simulink model "fft_biplex_test3"  (Simulink 7.6)
settings: Solver=ode45  StartTime=0.0  StopTime=5000  RelTol=1e-3
libraries: xbsIndex_r4 x1382, casper_library x82, monroe_library x27, xps_library x17, dspsigops x16, simulink x1
(part 3 of 13)

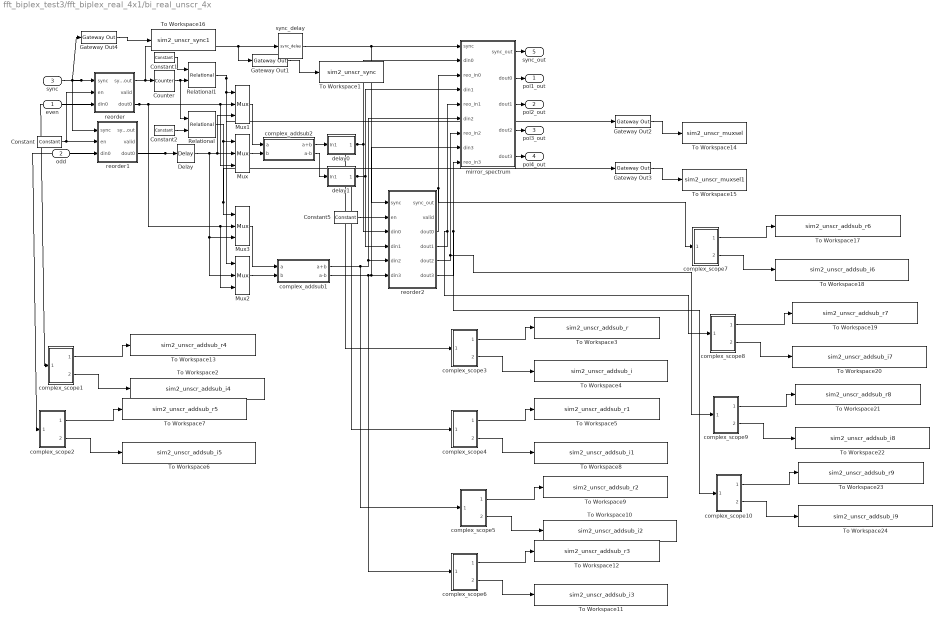
== system fft_biplex_test3/fft_biplex_real_4x1/bi_real_unscr_4x ==
  even : Inport
  odd : Inport  Port=2
  sync : Inport  Port=3
  Constant : xbsIndex_r4/Constant  arith_type=Boolean  const=1  n_bits=1  bin_pt=0  explicit_period=on  period=1  equ=P=C  opselect=C  inp2=PCIN>>17  opr=+  inp1=P  carry=CIN  dbl_ovrd=off  block_type=constant
      settings: block_version=9.1.01
  Constant1 : xbsIndex_r4/Constant  arith_type=Unsigned  const=2^(FFTSize-1)-1  n_bits=FFTSize  bin_pt=0  explicit_period=on  period=1  equ=P=C  opselect=C  inp2=PCIN>>17  opr=+  inp1=P  carry=CIN  dbl_ovrd=off  block_type=constant
      settings: block_version=9.1.01
  Constant2 : xbsIndex_r4/Constant  arith_type=Unsigned  const=2^FFTSize -1  n_bits=FFTSize  bin_pt=0  explicit_period=on  period=1  equ=P=C  opselect=C  inp2=PCIN>>17  opr=+  inp1=P  carry=CIN  dbl_ovrd=off  block_type=constant
      settings: block_version=9.1.01
  Constant5 : xbsIndex_r4/Constant  arith_type=Boolean  const=1  n_bits=1  bin_pt=0  explicit_period=on  period=1  equ=P=C  opselect=C  inp2=PCIN>>17  opr=+  inp1=P  carry=CIN  dbl_ovrd=off  block_type=constant
      settings: block_version=9.1.01
  Counter : xbsIndex_r4/Counter  cnt_type=Free Running  cnt_to=Inf  operation=Up  start_count=0  cnt_by_val=1  arith_type=Unsigned  n_bits=FFTSize  bin_pt=0  load_pin=off  rst=on  en=off  explicit_period=off  period=1  dbl_ovrd=off  use_behavioral_HDL=off  implementation=Fabric  use_rpm=on  block_type=counter
      settings: xl_area=[0, 0, 0, 0, 0, 0, 0]  block_version=9.1.01
  Delay : xbsIndex_r4/Delay  en=off  latency=1  dbl_ovrd=off  reg_retiming=off  block_type=delay
      settings: xl_area=[0, 0, 0, 0, 0, 0, 0]  block_version=9.1.01
  Gateway Out{1..4} (4 alike) : xbsIndex_r4/Gateway Out  hdl_port=on  timing_constraint=None  locs_specified=off  LOCs={}  block_type=gatewayout
      settings: infoedit="Gateway out block.  Converts Xilinx fixed point inputs into ouputs of type Simulink integer, double, or fixed point.<br><br>Hardware notes:  In hardware these blocks become top level output ports or are discarded, depending on how they are configured."  block_version=11.4
  Mux{,1..3} (4 alike) : xbsIndex_r4/Mux  inputs=2  en=off  latency=1  precision=Full  arith_type="Signed  (2's comp)"  n_bits=8  bin_pt=2  quantization=Truncate  overflow=Wrap  dbl_ovrd=off  block_type=mux
      settings: xl_area=[0, 0, 0, 0, 0, 0, 0]  block_version=9.1.01
  Relational : xbsIndex_r4/Relational  mode=a=b  en=off  latency=1  dbl_ovrd=off  block_type=relational
      settings: xl_area=[0, 0, 0, 0, 0, 0, 0]  block_version=9.1.01
  Relational1 : xbsIndex_r4/Relational  mode=a=b  en=off  latency=1  dbl_ovrd=off  block_type=relational
      settings: xl_area=[0, 0, 0, 0, 0, 0, 0]  block_version=9.1.01
  To Workspace1 : ToWorkspace  VariableName=sim2_unscr_sync  SampleTime=-1  SaveFormat=Structure
  To Workspace10 : ToWorkspace  VariableName=sim2_unscr_addsub_i2  SampleTime=-1  SaveFormat=Structure
  To Workspace11 : ToWorkspace  VariableName=sim2_unscr_addsub_i3  SampleTime=-1  SaveFormat=Structure
  To Workspace12 : ToWorkspace  VariableName=sim2_unscr_addsub_r3  SampleTime=-1  SaveFormat=Structure
  To Workspace13 : ToWorkspace  VariableName=sim2_unscr_addsub_r4  SampleTime=-1  SaveFormat=Structure
  To Workspace14 : ToWorkspace  VariableName=sim2_unscr_muxsel  SampleTime=-1  SaveFormat=Structure
  To Workspace15 : ToWorkspace  VariableName=sim2_unscr_muxsel1  SampleTime=-1  SaveFormat=Structure
  To Workspace16 : ToWorkspace  VariableName=sim2_unscr_sync1  SampleTime=-1  SaveFormat=Structure
  To Workspace17 : ToWorkspace  VariableName=sim2_unscr_addsub_r6  SampleTime=-1  SaveFormat=Structure
  To Workspace18 : ToWorkspace  VariableName=sim2_unscr_addsub_i6  SampleTime=-1  SaveFormat=Structure
  To Workspace19 : ToWorkspace  VariableName=sim2_unscr_addsub_r7  SampleTime=-1  SaveFormat=Structure
  To Workspace2 : ToWorkspace  VariableName=sim2_unscr_addsub_i4  SampleTime=-1  SaveFormat=Structure
  To Workspace20 : ToWorkspace  VariableName=sim2_unscr_addsub_i7  SampleTime=-1  SaveFormat=Structure
  To Workspace21 : ToWorkspace  VariableName=sim2_unscr_addsub_r8  SampleTime=-1  SaveFormat=Structure
  To Workspace22 : ToWorkspace  VariableName=sim2_unscr_addsub_i8  SampleTime=-1  SaveFormat=Structure
  To Workspace23 : ToWorkspace  VariableName=sim2_unscr_addsub_r9  SampleTime=-1  SaveFormat=Structure
  To Workspace24 : ToWorkspace  VariableName=sim2_unscr_addsub_i9  SampleTime=-1  SaveFormat=Structure
  To Workspace3 : ToWorkspace  VariableName=sim2_unscr_addsub_r  SampleTime=-1  SaveFormat=Structure
  To Workspace4 : ToWorkspace  VariableName=sim2_unscr_addsub_i  SampleTime=-1  SaveFormat=Structure
  To Workspace5 : ToWorkspace  VariableName=sim2_unscr_addsub_r1  SampleTime=-1  SaveFormat=Structure
  To Workspace6 : ToWorkspace  VariableName=sim2_unscr_addsub_i5  SampleTime=-1  SaveFormat=Structure
  To Workspace7 : ToWorkspace  VariableName=sim2_unscr_addsub_r5  SampleTime=-1  SaveFormat=Structure
  To Workspace8 : ToWorkspace  VariableName=sim2_unscr_addsub_i1  SampleTime=-1  SaveFormat=Structure
  To Workspace9 : ToWorkspace  VariableName=sim2_unscr_addsub_r2  SampleTime=-1  SaveFormat=Structure
  complex_addsub1 : Subsystem  mask(complex_addsub){BitWidth=input_bit_width, add_latency=add_latency}
      mask prompts: BitWidth "Bit Wdith"; add_latency "Add Latency"
      mask help:
      | Adds and subtracts the complex inputs.
      | If a = w + ix, b = y + iz then
      | a+b = (w+y)/2 + i(x-z)/2 and
      | a-b = (x+z)/2 + i(y-w)/2
  complex_addsub2 : Subsystem  mask(complex_addsub){BitWidth=input_bit_width, add_latency=add_latency}
      mask prompts: BitWidth "Bit Wdith"; add_latency "Add Latency"
      mask help:
      | Adds and subtracts the complex inputs.
      | If a = w + ix, b = y + iz then
      | a+b = (w+y)/2 + i(x-z)/2 and
      | a-b = (x+z)/2 + i(y-w)/2
  complex_scope1 : Subsystem
  complex_scope10 : Subsystem
  complex_scope2 : Subsystem
  complex_scope3 : Subsystem
  complex_scope4 : Subsystem
  complex_scope5 : Subsystem
  complex_scope6 : Subsystem
  complex_scope7 : Subsystem
  complex_scope8 : Subsystem
  complex_scope9 : Subsystem
  delay0 : Subsystem  AncestorBlock=casper_library/Delays/delay_bram  mask(delay_bram){DelayLen=2^(FFTSize-1), bram_latency=bram_latency, use_dsp48=off}
      mask prompts: DelayLen "Delay By:"; bram_latency "BRAM Latency"; use_dsp48 "Use DSP48"
      mask help: A delay block that uses BRAM for its storage.
      mask init:
      | if (DelayLen <= bram_latency)
      | 	error('delay value must be greater than BRAM Latency');
      | end
      | BitWidth = max(ceil(log2(DelayLen)), 2);
      | if strcmp(use_dsp48,'on'),
      |     set_param([gcb,'/Counter'], 'use_behavioral_HDL', 'off', ...
      |         'use_rpm', 'on', 'implementation', 'DSP48');
      | else, %default counter settings
      |         set_param([gcb,'/Counter'], 'use_behavioral_HDL', 'off', ...
      |         'use_rpm', 'off', 'implementation', 'Fabric');
      | end
      mask Help: eval('xlWeb(''http://casper.berkeley.edu/wiki/Delay_bram'')')
  delay1 : Subsystem  AncestorBlock=casper_library/Delays/delay_bram  mask(delay_bram){DelayLen=2^(FFTSize-1), bram_latency=bram_latency, use_dsp48=off}
      mask prompts: DelayLen "Delay By:"; bram_latency "BRAM Latency"; use_dsp48 "Use DSP48"
      mask help: A delay block that uses BRAM for its storage.
      mask init: same as fft_biplex_test3/fft_biplex_real_4x1/bi_real_unscr_4x/delay0
      mask Help: eval('xlWeb(''http://casper.berkeley.edu/wiki/Delay_bram'')')
  mirror_spectrum : Subsystem
  reorder : Subsystem  AncestorBlock=casper_library/Reorder/reorder  mask(reorder){map=getfield( getfield( get_param( gcb,'UserData' ), 'parameters'),'map'), n_inputs=1, bram_latency=3, map_latency=0, double_buffer=0}
      mask prompts: map "Output Order:"; n_inputs "Number of inputs"; bram_latency "BRAM Latency"; map_latency "Map Latency"; double_buffer "Double Buffer"
      mask init:
      | reorder_init(gcb, ...
      |     'map', map, ...
      |     'n_inputs', n_inputs, ...
      |     'bram_latency', bram_latency, ...
      |     'map_latency', map_latency, ...
      |     'double_buffer', double_buffer);
      settings: AttributesFormatString=order=2
  reorder1 : Subsystem  AncestorBlock=casper_library/Reorder/reorder  mask(reorder){map=getfield( getfield( get_param( gcb,'UserData' ), 'parameters'),'map'), n_inputs=1, bram_latency=3, map_latency=0, double_buffer=0}
      mask prompts: map "Output Order:"; n_inputs "Number of inputs"; bram_latency "BRAM Latency"; map_latency "Map Latency"; double_buffer "Double Buffer"
      mask init:
      | reorder_init(gcb, ...
      |     'map', map, ...
      |     'n_inputs', n_inputs, ...
      |     'bram_latency', bram_latency, ...
      |     'map_latency', map_latency, ...
      |     'double_buffer', double_buffer);
      settings: AttributesFormatString=order=2
  reorder2 : Subsystem  AncestorBlock=casper_library/Reorder/reorder  mask(reorder){map=getfield( getfield( get_param( gcb,'UserData' ), 'parameters'),'map'), n_inputs=4, bram_latency=3, map_latency=0, double_buffer=0}
      mask prompts: map "Output Order:"; n_inputs "Number of inputs"; bram_latency "BRAM Latency"; map_latency "Map Latency"; double_buffer "Double Buffer"
      mask init:
      | reorder_init(gcb, ...
      |     'map', map, ...
      |     'n_inputs', n_inputs, ...
      |     'bram_latency', bram_latency, ...
      |     'map_latency', map_latency, ...
      |     'double_buffer', double_buffer);
      settings: AttributesFormatString=order=2
  sync_delay : casper_library/Delays/sync_delay  SystemSampleTime=-1  DelayLen=2^(FFTSize-1) + 2*add_latency+1
  pol1_out : Outport
  pol2_out : Outport  Port=2
  pol3_out : Outport  Port=3
  pol4_out : Outport  Port=4
  sync_out : Outport  Port=5
  wires:
  reorder2/6(dout3) -> mirror_spectrum/9(reo_in3), complex_scope10/1(In1)
  reorder2/5(dout2) -> mirror_spectrum/7(reo_in2), complex_scope9/1(In1)
  reorder2/3(dout0) -> mirror_spectrum/3(reo_in0), complex_scope7/1(In1)
  reorder2/4(dout1) -> mirror_spectrum/5(reo_in1), complex_scope8/1(In1)
  mirror_spectrum/2(dout0) -> pol1_out/1
  mirror_spectrum/1(sync_out) -> sync_out/1
  sync_delay/1 -> mirror_spectrum/1(sync), reorder2/1(sync)
  Constant5/1 -> reorder2/2(en)
  delay0/1(Out1) -> mirror_spectrum/2(din0), reorder2/3(din0), complex_scope3/1(In1)
  delay1/1(Out1) -> mirror_spectrum/4(din1), reorder2/4(din1), complex_scope4/1(In1)
  complex_addsub1/1(a+b) -> mirror_spectrum/6(din2), reorder2/5(din2), complex_scope5/1(In1)
  complex_addsub1/2(a-b) -> mirror_spectrum/8(din3), reorder2/6(din3), complex_scope6/1(In1)
  complex_addsub2/2(a-b) -> delay1/1(In1)
  complex_addsub2/1(a+b) -> delay0/1(In1)
  Mux3/1 -> complex_addsub1/1(a)
  Mux2/1 -> complex_addsub1/2(b)
  Relational1/1 -> Mux1/1, Mux2/1, Gateway Out2/1
  Constant1/1 -> Relational1/1
  Counter/1 -> Relational1/2, Relational/1
  Constant2/1 -> Relational/2
  Mux1/1 -> complex_addsub2/1(a)
  sync/1 -> reorder1/1(sync), reorder/1(sync), Gateway Out4/1
  Constant/1 -> reorder1/2(en), reorder/2(en)
  reorder1/3(dout0) -> Delay/1, complex_scope2/1(In1)
  reorder/3(dout0) -> Mux3/2, Mux2/3, Mux1/2, Mux/3, complex_scope1/1(In1)
  reorder/1(sync_out) -> Counter/1, sync_delay/1, Gateway Out1/1
  Delay/1 -> Mux1/3, Mux/2, Mux3/3, Mux2/2
  Mux/1 -> complex_addsub2/2(b)
  Relational/1 -> Mux/1, Mux3/1, Gateway Out3/1
  even/1 -> reorder/3(din0)
  odd/1 -> reorder1/3(din0)
  mirror_spectrum/3(dout1) -> pol2_out/1
  mirror_spectrum/4(dout2) -> pol3_out/1
  mirror_spectrum/5(dout3) -> pol4_out/1
  complex_scope3/1(Real) -> To Workspace3/1
  complex_scope3/2(Imag) -> To Workspace4/1
  complex_scope4/1(Real) -> To Workspace5/1
  complex_scope4/2(Imag) -> To Workspace8/1
  complex_scope5/1(Real) -> To Workspace9/1
  complex_scope5/2(Imag) -> To Workspace10/1
  complex_scope6/1(Real) -> To Workspace12/1
  complex_scope6/2(Imag) -> To Workspace11/1
  Gateway Out1/1 -> To Workspace1/1
  Gateway Out2/1 -> To Workspace14/1
  Gateway Out3/1 -> To Workspace15/1
  Gateway Out4/1 -> To Workspace16/1
  complex_scope1/1(Real) -> To Workspace13/1
  complex_scope1/2(Imag) -> To Workspace2/1
  complex_scope2/1(Real) -> To Workspace7/1
  complex_scope2/2(Imag) -> To Workspace6/1
  complex_scope7/1(Real) -> To Workspace17/1
  complex_scope7/2(Imag) -> To Workspace18/1
  complex_scope8/1(Real) -> To Workspace19/1
  complex_scope8/2(Imag) -> To Workspace20/1
  complex_scope9/1(Real) -> To Workspace21/1
  complex_scope9/2(Imag) -> To Workspace22/1
  complex_scope10/1(Real) -> To Workspace23/1
  complex_scope10/2(Imag) -> To Workspace24/1

== system fft_biplex_test3/fft_biplex_real_4x1/biplex_core ==
  pol1 : Inport
  pol2 : Inport  Port=2
  sync : Inport  Port=3
  shift : Inport  Port=4
  Constant : xbsIndex_r4/Constant  arith_type=Boolean  const=0  n_bits=1  bin_pt=1  explicit_period=off  period=1  equ=P=C  opselect=C  inp2=PCIN>>17  opr=+  inp1=P  carry=CIN  dbl_ovrd=off  block_type=constant
  To Workspace1 : ToWorkspace  VariableName=sim2_stg4_r  SampleTime=-1  SaveFormat=Structure
  To Workspace10 : ToWorkspace  VariableName=sim2_stg3_r  SampleTime=-1  SaveFormat=Structure
  To Workspace11 : ToWorkspace  VariableName=sim2_stg3_i  SampleTime=-1  SaveFormat=Structure
  To Workspace12 : ToWorkspace  VariableName=sim2_stg2_i1  SampleTime=-1  SaveFormat=Structure
  To Workspace2 : ToWorkspace  VariableName=sim2_stg4_i  SampleTime=-1  SaveFormat=Structure
  To Workspace3 : ToWorkspace  VariableName=sim2_stg4_r1  SampleTime=-1  SaveFormat=Structure
  To Workspace4 : ToWorkspace  VariableName=sim2_stg3_r1  SampleTime=-1  SaveFormat=Structure
  To Workspace5 : ToWorkspace  VariableName=sim2_stg3_i1  SampleTime=-1  SaveFormat=Structure
  To Workspace6 : ToWorkspace  VariableName=sim2_stg4_i1  SampleTime=-1  SaveFormat=Structure
  To Workspace7 : ToWorkspace  VariableName=sim2_stg2_r  SampleTime=-1  SaveFormat=Structure
  To Workspace8 : ToWorkspace  VariableName=sim2_stg2_i  SampleTime=-1  SaveFormat=Structure
  To Workspace9 : ToWorkspace  VariableName=sim2_stg2_r1  SampleTime=-1  SaveFormat=Structure
  complex_scope1 : Subsystem
  complex_scope2 : Subsystem
  complex_scope3 : Subsystem
  complex_scope4 : Subsystem
  complex_scope5 : Subsystem
  complex_scope6 : Subsystem
  fft_stage_1 : Subsystem  AncestorBlock=casper_library/FFTs/fft_stage_n  mask(fft_stage_n){FFTSize=5, FFTStage=1, input_bit_width=8, coeff_bit_width=18, delays_bram=on, coeffs_bram=off, MaxCoeffNum=20, quantization=Truncate, overflow=Wrap, add_latency=2, mult_latency=3, bram_latency=3, arch=Virtex5, opt_target=Logic, use_hdl=on, use_embedded=off, dsp48_adders=on, shift=1, output_bit_width=18}
      mask prompts: FFTSize "Size of FFT: (2^? pnts)"; FFTStage "Stage of FFT:"; input_bit_width "Input Bit Width:"; coeff_bit_width "Coefficient Bit Width"; delays_bram "Implement Delays in BRAM:"; coeffs_bram "Store Coefficients in BRAM:"; MaxCoeffNum "Maximum Coefficient Depth: (2^?)"; quantization "Quantization Behavior"; overflow "Overflow Behavior"; add_latency "Add Latency"; mult_latency "Mult Latency"; bram_latency "BRAM Latency"; arch "Architecture"; opt_target "Optimisation target"; use_hdl "Use behavioural HDL for mutlipliers"; use_embedded "Use embedded multipliers"; dsp48_adders "Use DSP48s for adders"; shift "Downshift binary point?"; output_bit_width "Output Bit Width"
      mask init:
      | fft_stage_n_init(gcb,...
      |     'FFTSize', FFTSize,...
      |     'FFTStage', FFTStage,...
      |     'input_bit_width', input_bit_width,...
      |     'output_bit_width', output_bit_width,...
      |     'coeff_bit_width', coeff_bit_width,...
      |     'delays_bram', delays_bram,...
      |     'coeffs_bram', coeffs_bram,...
      |     'MaxCoeffNum', MaxCoeffNum,...
      |     'quantization', quantization,...
      |     'overflow', overflow,...
      |     'add_latency', add_latency,...
      |     'mult_latency', mult_latency,...
      |     'bram_latency', bram_latency,...
      |     'arch', arch, ...
      |     'opt_target', opt_target, ...
      |     'use_hdl', use_hdl,...
      |     'use_embedded', use_embedded, ...
      |     'dsp48_adders', dsp48_adders, ...
      |     'output_bit_width', output_bit_width, ...
      |     'shift', shift );
      settings: AttributesFormatString=|
      | FFTSize=5, FFTStage=1,
      |  coeffs_bram=off,
      |  delays_bram=on
      mask StyleString: edit,edit,edit,edit,checkbox,checkbox,edit,popup(Truncate|Round  (unbiased: +/- Inf)|Round  (unbiased: Even Values)),popup(Wrap|Saturate|Error),edit,edit,edit,popup(Virtex2Pro|Virtex5),popup(Logic|Multipliers),checkbox,checkbox,checkbox,edit,edit
      mask CallbackString:
      | ||||||||||||||use_hdl = get_param(gcb,'use_hdl');
      | visibs = get_param(gcb, 'MaskVisibilities');
      | if( strcmp(use_hdl,'on')),
      |     visibs{16} = 'off';
      | else,
      |     visibs{16} = 'on';
      | end
      |     set_param(gcb, 'MaskVisibilities',visibs);||||
  fft_stage_2 : Subsystem  AncestorBlock=casper_library/FFTs/fft_stage_n  mask(fft_stage_n){FFTSize=5, FFTStage=2, input_bit_width=18, coeff_bit_width=18, delays_bram=on, coeffs_bram=off, MaxCoeffNum=20, quantization=Truncate, overflow=Wrap, add_latency=2, mult_latency=3, bram_latency=3, arch=Virtex5, opt_target=Logic, use_hdl=on, use_embedded=off, dsp48_adders=on, shift=1, output_bit_width=18}
      mask prompts: FFTSize "Size of FFT: (2^? pnts)"; FFTStage "Stage of FFT:"; input_bit_width "Input Bit Width:"; coeff_bit_width "Coefficient Bit Width"; delays_bram "Implement Delays in BRAM:"; coeffs_bram "Store Coefficients in BRAM:"; MaxCoeffNum "Maximum Coefficient Depth: (2^?)"; quantization "Quantization Behavior"; overflow "Overflow Behavior"; add_latency "Add Latency"; mult_latency "Mult Latency"; bram_latency "BRAM Latency"; arch "Architecture"; opt_target "Optimisation target"; use_hdl "Use behavioural HDL for mutlipliers"; use_embedded "Use embedded multipliers"; dsp48_adders "Use DSP48s for adders"; shift "Downshift binary point?"; output_bit_width "Output Bit Width"
      mask init: same as fft_biplex_test3/fft_biplex_real_4x1/biplex_core/fft_stage_1
      settings: AttributesFormatString=|
      | FFTSize=5, FFTStage=2,
      |  coeffs_bram=off,
      |  delays_bram=on
      mask StyleString: edit,edit,edit,edit,checkbox,checkbox,edit,popup(Truncate|Round  (unbiased: +/- Inf)|Round  (unbiased: Even Values)),popup(Wrap|Saturate|Error),edit,edit,edit,popup(Virtex2Pro|Virtex5),popup(Logic|Multipliers),checkbox,checkbox,checkbox,edit,edit
      mask CallbackString:
      | ||||||||||||||use_hdl = get_param(gcb,'use_hdl');
      | visibs = get_param(gcb, 'MaskVisibilities');
      | if( strcmp(use_hdl,'on')),
      |     visibs{16} = 'off';
      | else,
      |     visibs{16} = 'on';
      | end
      |     set_param(gcb, 'MaskVisibilities',visibs);||||
  fft_stage_3 : Subsystem  AncestorBlock=casper_library/FFTs/fft_stage_n  mask(fft_stage_n){FFTSize=5, FFTStage=3, input_bit_width=18, coeff_bit_width=18, delays_bram=off, coeffs_bram=off, MaxCoeffNum=20, quantization=Truncate, overflow=Wrap, add_latency=2, mult_latency=3, bram_latency=3, arch=Virtex5, opt_target=Logic, use_hdl=on, use_embedded=off, dsp48_adders=on, shift=1, output_bit_width=18}
      mask prompts: FFTSize "Size of FFT: (2^? pnts)"; FFTStage "Stage of FFT:"; input_bit_width "Input Bit Width:"; coeff_bit_width "Coefficient Bit Width"; delays_bram "Implement Delays in BRAM:"; coeffs_bram "Store Coefficients in BRAM:"; MaxCoeffNum "Maximum Coefficient Depth: (2^?)"; quantization "Quantization Behavior"; overflow "Overflow Behavior"; add_latency "Add Latency"; mult_latency "Mult Latency"; bram_latency "BRAM Latency"; arch "Architecture"; opt_target "Optimisation target"; use_hdl "Use behavioural HDL for mutlipliers"; use_embedded "Use embedded multipliers"; dsp48_adders "Use DSP48s for adders"; shift "Downshift binary point?"; output_bit_width "Output Bit Width"
      mask init: same as fft_biplex_test3/fft_biplex_real_4x1/biplex_core/fft_stage_1
      settings: AttributesFormatString=|
      | FFTSize=5, FFTStage=3,
      |  coeffs_bram=off,
      |  delays_bram=off
      mask StyleString: edit,edit,edit,edit,checkbox,checkbox,edit,popup(Truncate|Round  (unbiased: +/- Inf)|Round  (unbiased: Even Values)),popup(Wrap|Saturate|Error),edit,edit,edit,popup(Virtex2Pro|Virtex5),popup(Logic|Multipliers),checkbox,checkbox,checkbox,edit,edit
      mask CallbackString:
      | ||||||||||||||use_hdl = get_param(gcb,'use_hdl');
      | visibs = get_param(gcb, 'MaskVisibilities');
      | if( strcmp(use_hdl,'on')),
      |     visibs{16} = 'off';
      | else,
      |     visibs{16} = 'on';
      | end
      |     set_param(gcb, 'MaskVisibilities',visibs);||||
  fft_stage_4 : Subsystem  AncestorBlock=casper_library/FFTs/fft_stage_n  mask(fft_stage_n){FFTSize=5, FFTStage=4, input_bit_width=18, coeff_bit_width=18, delays_bram=off, coeffs_bram=off, MaxCoeffNum=20, quantization=Truncate, overflow=Wrap, add_latency=2, mult_latency=3, bram_latency=3, arch=Virtex5, opt_target=Logic, use_hdl=on, use_embedded=off, dsp48_adders=on, shift=1, output_bit_width=18}
      mask prompts: FFTSize "Size of FFT: (2^? pnts)"; FFTStage "Stage of FFT:"; input_bit_width "Input Bit Width:"; coeff_bit_width "Coefficient Bit Width"; delays_bram "Implement Delays in BRAM:"; coeffs_bram "Store Coefficients in BRAM:"; MaxCoeffNum "Maximum Coefficient Depth: (2^?)"; quantization "Quantization Behavior"; overflow "Overflow Behavior"; add_latency "Add Latency"; mult_latency "Mult Latency"; bram_latency "BRAM Latency"; arch "Architecture"; opt_target "Optimisation target"; use_hdl "Use behavioural HDL for mutlipliers"; use_embedded "Use embedded multipliers"; dsp48_adders "Use DSP48s for adders"; shift "Downshift binary point?"; output_bit_width "Output Bit Width"
      mask init: same as fft_biplex_test3/fft_biplex_real_4x1/biplex_core/fft_stage_1
      settings: AttributesFormatString=|
      | FFTSize=5, FFTStage=4,
      |  coeffs_bram=off,
      |  delays_bram=off
      mask StyleString: edit,edit,edit,edit,checkbox,checkbox,edit,popup(Truncate|Round  (unbiased: +/- Inf)|Round  (unbiased: Even Values)),popup(Wrap|Saturate|Error),edit,edit,edit,popup(Virtex2Pro|Virtex5),popup(Logic|Multipliers),checkbox,checkbox,checkbox,edit,edit
      mask CallbackString:
      | ||||||||||||||use_hdl = get_param(gcb,'use_hdl');
      | visibs = get_param(gcb, 'MaskVisibilities');
      | if( strcmp(use_hdl,'on')),
      |     visibs{16} = 'off';
      | else,
      |     visibs{16} = 'on';
      | end
      |     set_param(gcb, 'MaskVisibilities',visibs);||||
  fft_stage_5 : Subsystem  AncestorBlock=casper_library/FFTs/fft_stage_n  mask(fft_stage_n){FFTSize=5, FFTStage=5, input_bit_width=18, coeff_bit_width=18, delays_bram=off, coeffs_bram=off, MaxCoeffNum=20, quantization=Truncate, overflow=Wrap, add_latency=2, mult_latency=3, bram_latency=3, arch=Virtex5, opt_target=Logic, use_hdl=on, use_embedded=off, dsp48_adders=on, shift=1, output_bit_width=18}
      mask prompts: FFTSize "Size of FFT: (2^? pnts)"; FFTStage "Stage of FFT:"; input_bit_width "Input Bit Width:"; coeff_bit_width "Coefficient Bit Width"; delays_bram "Implement Delays in BRAM:"; coeffs_bram "Store Coefficients in BRAM:"; MaxCoeffNum "Maximum Coefficient Depth: (2^?)"; quantization "Quantization Behavior"; overflow "Overflow Behavior"; add_latency "Add Latency"; mult_latency "Mult Latency"; bram_latency "BRAM Latency"; arch "Architecture"; opt_target "Optimisation target"; use_hdl "Use behavioural HDL for mutlipliers"; use_embedded "Use embedded multipliers"; dsp48_adders "Use DSP48s for adders"; shift "Downshift binary point?"; output_bit_width "Output Bit Width"
      mask init: same as fft_biplex_test3/fft_biplex_real_4x1/biplex_core/fft_stage_1
      settings: AttributesFormatString=|
      | FFTSize=5, FFTStage=5,
      |  coeffs_bram=off,
      |  delays_bram=off
      mask StyleString: edit,edit,edit,edit,checkbox,checkbox,edit,popup(Truncate|Round  (unbiased: +/- Inf)|Round  (unbiased: Even Values)),popup(Wrap|Saturate|Error),edit,edit,edit,popup(Virtex2Pro|Virtex5),popup(Logic|Multipliers),checkbox,checkbox,checkbox,edit,edit
      mask CallbackString:
      | ||||||||||||||use_hdl = get_param(gcb,'use_hdl');
      | visibs = get_param(gcb, 'MaskVisibilities');
      | if( strcmp(use_hdl,'on')),
      |     visibs{16} = 'off';
      | else,
      |     visibs{16} = 'on';
      | end
      |     set_param(gcb, 'MaskVisibilities',visibs);||||
  out1 : Outport
  out2 : Outport  Port=2
  of : Outport  Port=3
  sync_out : Outport  Port=4
  wires:
  sync/1 -> fft_stage_1/4(sync)
  Constant/1 -> fft_stage_1/3(of_in)
  pol2/1 -> fft_stage_1/2(in2)
  pol1/1 -> fft_stage_1/1(in1)
  fft_stage_5/4(sync_out) -> sync_out/1
  fft_stage_5/3(of) -> of/1
  fft_stage_5/2(out2) -> out2/1
  fft_stage_5/1(out1) -> out1/1
  fft_stage_4/4(sync_out) -> fft_stage_5/4(sync)
  fft_stage_4/3(of) -> fft_stage_5/3(of_in)
  fft_stage_4/2(out2) -> fft_stage_5/2(in2), complex_scope2/1(In1)
  fft_stage_4/1(out1) -> fft_stage_5/1(in1), complex_scope1/1(In1)
  fft_stage_3/4(sync_out) -> fft_stage_4/4(sync)
  fft_stage_3/3(of) -> fft_stage_4/3(of_in)
  fft_stage_3/2(out2) -> fft_stage_4/2(in2), complex_scope3/1(In1)
  fft_stage_3/1(out1) -> fft_stage_4/1(in1), complex_scope4/1(In1)
  fft_stage_2/4(sync_out) -> fft_stage_3/4(sync)
  fft_stage_2/3(of) -> fft_stage_3/3(of_in)
  fft_stage_2/2(out2) -> fft_stage_3/2(in2), complex_scope6/1(In1)
  fft_stage_2/1(out1) -> fft_stage_3/1(in1), complex_scope5/1(In1)
  shift/1 -> fft_stage_1/5(shift), fft_stage_5/5(shift), fft_stage_4/5(shift), fft_stage_3/5(shift), fft_stage_2/5(shift)
  fft_stage_1/4(sync_out) -> fft_stage_2/4(sync)
  fft_stage_1/3(of) -> fft_stage_2/3(of_in)
  fft_stage_1/2(out2) -> fft_stage_2/2(in2)
  fft_stage_1/1(out1) -> fft_stage_2/1(in1)
  complex_scope4/1(Real) -> To Workspace10/1
  complex_scope4/2(Imag) -> To Workspace11/1
  complex_scope1/1(Real) -> To Workspace1/1
  complex_scope1/2(Imag) -> To Workspace2/1
  complex_scope3/1(Real) -> To Workspace4/1
  complex_scope3/2(Imag) -> To Workspace5/1
  complex_scope2/1(Real) -> To Workspace3/1
  complex_scope2/2(Imag) -> To Workspace6/1
  complex_scope5/1(Real) -> To Workspace7/1
  complex_scope5/2(Imag) -> To Workspace8/1
  complex_scope6/1(Real) -> To Workspace9/1
  complex_scope6/2(Imag) -> To Workspace12/1

== system fft_biplex_test3/fft_biplex_real_4x1/ri_to_c ==
  re : Inport
  im : Inport  Port=2
  Concat : xbsIndex_r4/Concat  num_inputs=2  dbl_ovrd=off  block_type=concat
      settings: block_version=9.1.01
  Reinterpret : xbsIndex_r4/Reinterpret  force_arith_type=on  arith_type=Unsigned  force_bin_pt=on  bin_pt=0  block_type=reinterpret
      settings: infoedit="Changes signal type without altering the binary representation.   You can changed the signal between signed and unsigned, and relocate the binary point.<P><P>Hardware notes: In hardware this block costs nothing.<P><P>Example:  Suppose the input is 6 bits wide, signed, with 2 fractional bits, and the output is forced to unsigned with 0 fractional bits.  Then an input of -2.0 (1110.00 in binary 2's complement) becomes an output of 56 (111000 in binary)."  block_version=9.1.01
  Reinterpret1 : xbsIndex_r4/Reinterpret  force_arith_type=on  arith_type=Unsigned  force_bin_pt=on  bin_pt=0  block_type=reinterpret
      settings: infoedit="Changes signal type without altering the binary representation.   You can changed the signal between signed and unsigned, and relocate the binary point.<P><P>Hardware notes: In hardware this block costs nothing.<P><P>Example:  Suppose the input is 6 bits wide, signed, with 2 fractional bits, and the output is forced to unsigned with 0 fractional bits.  Then an input of -2.0 (1110.00 in binary 2's complement) becomes an output of 56 (111000 in binary)."  block_version=9.1.01
  c : Outport
  wires:
  im/1 -> Reinterpret1/1
  Concat/1 -> c/1
  re/1 -> Reinterpret/1
  Reinterpret1/1 -> Concat/2
  Reinterpret/1 -> Concat/1

== system fft_biplex_test3/fft_biplex_real_4x1/ri_to_c1 ==
  re : Inport
  im : Inport  Port=2
  Concat : xbsIndex_r4/Concat  num_inputs=2  dbl_ovrd=off  block_type=concat
      settings: block_version=9.1.01
  Reinterpret : xbsIndex_r4/Reinterpret  force_arith_type=on  arith_type=Unsigned  force_bin_pt=on  bin_pt=0  block_type=reinterpret
      settings: infoedit="Changes signal type without altering the binary representation.   You can changed the signal between signed and unsigned, and relocate the binary point.<P><P>Hardware notes: In hardware this block costs nothing.<P><P>Example:  Suppose the input is 6 bits wide, signed, with 2 fractional bits, and the output is forced to unsigned with 0 fractional bits.  Then an input of -2.0 (1110.00 in binary 2's complement) becomes an output of 56 (111000 in binary)."  block_version=9.1.01
  Reinterpret1 : xbsIndex_r4/Reinterpret  force_arith_type=on  arith_type=Unsigned  force_bin_pt=on  bin_pt=0  block_type=reinterpret
      settings: infoedit="Changes signal type without altering the binary representation.   You can changed the signal between signed and unsigned, and relocate the binary point.<P><P>Hardware notes: In hardware this block costs nothing.<P><P>Example:  Suppose the input is 6 bits wide, signed, with 2 fractional bits, and the output is forced to unsigned with 0 fractional bits.  Then an input of -2.0 (1110.00 in binary 2's complement) becomes an output of 56 (111000 in binary)."  block_version=9.1.01
  c : Outport
  wires:
  im/1 -> Reinterpret1/1
  Concat/1 -> c/1
  re/1 -> Reinterpret/1
  Reinterpret1/1 -> Concat/2
  Reinterpret/1 -> Concat/1

== system fft_biplex_test3/FFT_Biplex_4x/biplex_4x_unscr/dual_bit_reverse ==
  sync : Inport
  din0 : Inport  Port=2
  din1 : Inport  Port=3
  Concat1 : xbsIndex_r4/Concat  num_inputs=2  dbl_ovrd=off  block_type=concat
  Concat2 : xbsIndex_r4/Concat  num_inputs=2  dbl_ovrd=off  block_type=concat
  Constant : xbsIndex_r4/Constant  arith_type=Boolean  const=1  n_bits=1  bin_pt=0  explicit_period=on  period=1  equ=P=C  opselect=C  inp2=PCIN>>17  opr=+  inp1=P  carry=CIN  dbl_ovrd=off  block_type=constant
  Constant1 : xbsIndex_r4/Constant  arith_type=Boolean  const=0  n_bits=1  bin_pt=0  explicit_period=on  period=1  equ=P=C  opselect=C  inp2=PCIN>>17  opr=+  inp1=P  carry=CIN  dbl_ovrd=off  block_type=constant
  Constant5 : xbsIndex_r4/Constant  arith_type=Boolean  const=1  n_bits=1  bin_pt=0  explicit_period=on  period=1  equ=P=C  opselect=C  inp2=PCIN>>17  opr=+  inp1=P  carry=CIN  dbl_ovrd=off  block_type=constant
  Counter : xbsIndex_r4/Counter  cnt_type=Free Running  cnt_to=1023  operation=Up  start_count=0  cnt_by_val=1  arith_type=Unsigned  n_bits=10  bin_pt=0  load_pin=off  rst=on  en=off  explicit_period=on  period=1  dbl_ovrd=off  use_behavioral_HDL=off  implementation=Fabric  use_rpm=off  block_type=counter
  Counter1 : xbsIndex_r4/Counter  cnt_type=Free Running  cnt_to=1023  operation=Down  start_count=1023  cnt_by_val=1  arith_type=Unsigned  n_bits=10  bin_pt=0  load_pin=off  rst=on  en=off  explicit_period=on  period=1  dbl_ovrd=off  use_behavioral_HDL=off  implementation=Fabric  use_rpm=off  block_type=counter
  Dual Port RAM : xbsIndex_r4/Dual Port RAM  depth=1024  initVector=sin(pi*(0:15)/16)  distributed_mem=Block RAM  init_a=0  init_b=0  rst_a=off  rst_b=off  en_a=off  en_b=off  latency=2  write_mode_A=Read Before Write  write_mode_B=Read Before Write  dbl_ovrd=off  optimize=Area  use_rpm=on  block_type=dpram
  Inverter : xbsIndex_r4/Inverter  en=off  latency=0  dbl_ovrd=off  block_type=inv
  Mux : xbsIndex_r4/Mux  inputs=2  en=off  latency=0  precision=Full  arith_type=Unsigned  n_bits=16  bin_pt=14  quantization=Truncate  overflow=Wrap  dbl_ovrd=off  block_type=mux
  Mux1 : xbsIndex_r4/Mux  inputs=2  en=off  latency=0  precision=Full  arith_type=Unsigned  n_bits=16  bin_pt=14  quantization=Truncate  overflow=Wrap  dbl_ovrd=off  block_type=mux
  Slice1 : xbsIndex_r4/Slice  nbits=1  boolean_output=off  mode=Upper Bit Location + Width  bit1=0  base1=MSB of Input  bit0=0  base0=LSB of Input  dbl_ovrd=off  block_type=slice
  Slice2 : xbsIndex_r4/Slice  nbits=9  boolean_output=off  mode=Lower Bit Location + Width  bit1=0  base1=MSB of Input  bit0=0  base0=LSB of Input  dbl_ovrd=off  block_type=slice
  Slice3 : xbsIndex_r4/Slice  nbits=1  boolean_output=off  mode=Upper Bit Location + Width  bit1=0  base1=MSB of Input  bit0=0  base0=LSB of Input  dbl_ovrd=off  block_type=slice
  Slice4 : xbsIndex_r4/Slice  nbits=9  boolean_output=off  mode=Lower Bit Location + Width  bit1=0  base1=MSB of Input  bit0=0  base0=LSB of Input  dbl_ovrd=off  block_type=slice
  bit_reverse_1 : Subsystem
  bit_reverse_2 : Subsystem
  delay_din0 : xbsIndex_r4/Delay  en=off  latency=0  dbl_ovrd=off  reg_retiming=off  block_type=delay
  delay_din1 : xbsIndex_r4/Delay  en=off  latency=0  dbl_ovrd=off  reg_retiming=off  block_type=delay
  post_sync_delay : xbsIndex_r4/Delay  en=off  latency=2  dbl_ovrd=off  reg_retiming=off  block_type=delay
  post_sync_delay1 : xbsIndex_r4/Delay  en=off  latency=0  dbl_ovrd=off  reg_retiming=off  block_type=delay
  sync_delay_fast : monroe_library/sync_delay_fast  SystemSampleTime=-1  delay_len=512
  sync_out : Outport
  dout0 : Outport  Port=2
  dout1 : Outport  Port=3
  wires:
  Constant1/1 -> Concat1/1
  Constant5/1 -> Concat2/1
  Concat2/1 -> Dual Port RAM/1
  Concat1/1 -> Dual Port RAM/4
  Dual Port RAM/1 -> dout0/1
  Dual Port RAM/2 -> dout1/1
  Mux/1 -> Concat2/2
  Mux1/1 -> Concat1/2
  Slice3/1 -> Inverter/1
  din0/1 -> delay_din0/1
  delay_din0/1 -> Dual Port RAM/2
  din1/1 -> delay_din1/1
  delay_din1/1 -> Dual Port RAM/5
  post_sync_delay/1 -> sync_out/1
  sync/1 -> post_sync_delay1/1
  sync_delay_fast/1 -> post_sync_delay/1
  bit_reverse_1/1(out) -> Mux/3
  Slice4/1 -> bit_reverse_2/1(in)  "xlsub3_Slice4_out1"
  bit_reverse_2/1(out) -> Mux1/3
  post_sync_delay1/1 -> Counter/1, Counter1/1, sync_delay_fast/1
  Counter1/1 -> Slice3/1, Slice4/1
  Slice2/1 -> Mux/2, Mux1/2, bit_reverse_1/1(in)
  Slice1/1 -> Mux/1, Mux1/1
  Counter/1 -> Slice1/1, Slice2/1
  Constant/1 -> Dual Port RAM/3, Dual Port RAM/6
